simulink model "Half_car_model_susp_bump_tyre"  (R2025b)
settings: Solver=VariableStepAuto  StartTime=0.0  StopTime=10.0  RelTol=1e-3
undefined symbols (not defined in the file or in its folder): bump_t_dist, delta0, Ks, p, r0, u0, x0, x0_lin
libraries: simulink x1

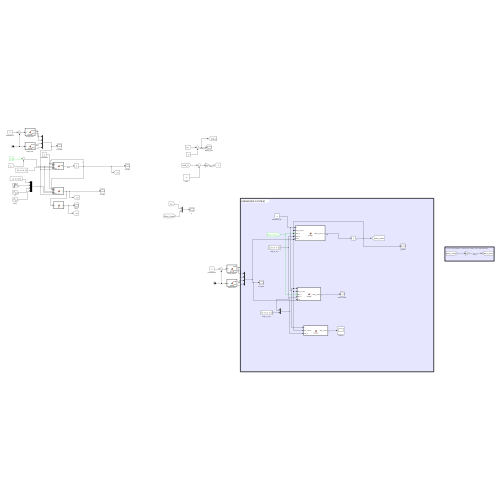
[thumbnail: Simulink's stored preview of the top-level diagram]
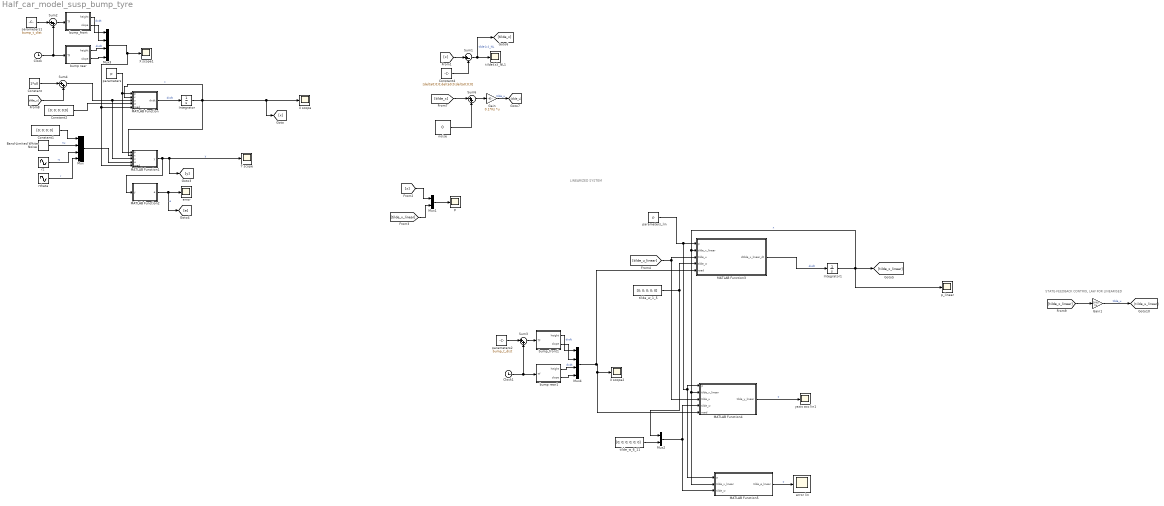
== system Half_car_model_susp_bump_tyre ==
  note: LINEARIZED SYSTEM
  note: STATE-FEEDBACK CONTROL LAW FOR LINEARISED
  " error lin" : Scope
      settings: ActiveDisplayYMinimum=-1  ActiveDisplayYMaximum=1  DataLoggingVariableName=ScopeData5
  Band-Limited White Noise : simulink/Sources/Band-Limited White Noise  Cov="1*[0.00001*1e-2; 0.00001*1e-2;  0.00001*1e-2; 0.00001*1e-2; 0.00001*1e-2]"  Ts=1e-2  seed=[23341; 31826; 11111; 81818; 00001]
  Clock : Clock
  Clock1 : Clock
  Constant : Constant  Value=1*u0
  Constant1 : Constant  Value=[0; 0; 0; 0]
  Constant2 : Constant  Value=[0; 0; 0; 0;0]
  Constant4 : Constant  Value=[delta0;0;0;delta0;0;delta0;0;0]
  Gain : Gain  Gain=0.1*Ks  Multiplication=Matrix(K*u)
  Gain1 : Gain  Gain=1*Ks  Multiplication=Matrix(K*u)
  Integrator : Integrator  InitialCondition=x0
  Integrator1 : Integrator  InitialCondition=x0_lin
  MATLAB Function : MATLAB Function  TreatAsAtomicUnit=on
  MATLAB Function1 : MATLAB Function  TreatAsAtomicUnit=on
  MATLAB Function2 : MATLAB Function  TreatAsAtomicUnit=on
  MATLAB Function3 : MATLAB Function  TreatAsAtomicUnit=on
  MATLAB Function4 : MATLAB Function  TreatAsAtomicUnit=on
  MATLAB Function5 : MATLAB Function  TreatAsAtomicUnit=on
  Mux : Mux
  Mux1 : Mux  Inputs=2
  Mux2 : Mux  Inputs=2
  Mux3 : Mux
  Mux4 : Mux
  Sum1 : Sum  Inputs=|+-
  Sum{2..4,6} (4 alike) : Sum  Inputs=|++
  X scope : Scope
      settings: ActiveDisplayYMinimum=-2.9269551656829207  ActiveDisplayYMaximum=2.5364123096854247  DataLoggingVariableName=ScopeData2
  X scope1 : Scope
      settings: ActiveDisplayYMinimum=-0.062253584416077451  ActiveDisplayYMaximum=0.56028225974469714
  X scope2 : Scope
      settings: ActiveDisplayYMinimum=-2.6804502153599614  ActiveDisplayYMaximum=1.9213273662141332  DataLoggingVariableName=ScopeData9
  Y scope : Scope
      settings: ActiveDisplayYMinimum=-4.5656742824498968  ActiveDisplayYMaximum=4.3230780985024841  DataLoggingVariableName=ScopeData3
  bump rear : MATLAB Function  TreatAsAtomicUnit=on
  bump rear1 : MATLAB Function  TreatAsAtomicUnit=on
  bump_front : MATLAB Function  TreatAsAtomicUnit=on
  bump_front1 : MATLAB Function  TreatAsAtomicUnit=on
  "error " : Scope
      settings: ActiveDisplayYMinimum=-0.92138  ActiveDisplayYMaximum=0.76934  DataLoggingVariableName=ScopeData6
  noise : Constant  Value=0
  p : Scope
      settings: ActiveDisplayYMinimum=-2.11909  ActiveDisplayYMaximum=2.06603
  p_linear : Scope
      settings: ActiveDisplayYMinimum=-1.85296  ActiveDisplayYMaximum=0.95967  DataLoggingVariableName=ScopeData7
  parameters : Constant  Value=p
  parameters1 : Constant  Value=bump_t_dist
  parameters2 : Constant  Value=bump_t_dist
  parameters_lin : Constant  Value=p
  rtheta : Sin  Amplitude=0  Bias=r0  Frequency=0  SampleTime=0
  rz : Sin  Amplitude=0  Bias=r0  Frequency=0  SampleTime=0
  tilde_w_1_5 : Constant  Value=[0; 0; 0; 0; 0]
  tilde_w_6_11 : Constant  Value=[0; 0; 0; 0; 0; 0]
  "tilde{x}_NL1" : Scope
      settings: ActiveDisplayYMinimum=-4.93552  ActiveDisplayYMaximum=2.55492  DataLoggingVariableName=ScopeData4
  yaxis acc lin1 : Scope
      settings: ActiveDisplayYMinimum=-1  ActiveDisplayYMaximum=1  DataLoggingVariableName=ScopeData8
  wires:
  bump rear/1(height) -> Mux3/3  "dxdt"
  Clock/1 -> Sum2/2, bump rear/1(Tf)
  bump_front/2(slope) -> Mux3/2
  bump rear/2(slope) -> Mux3/4
  Sum2/1 -> bump_front/1(Tf)
  parameters1/1 -> Sum2/1
  Mux3/1 -> MATLAB Function1/5(road), MATLAB Function/5(road), X scope1/1
  bump_front/1(height) -> Mux3/1  "dxdt"
  Constant/1 -> Sum4/1
  [tilde_u] -> Sum4/2
  Sum4/1 -> MATLAB Function1/3(u), MATLAB Function/3(u)
  Constant2/1 -> MATLAB Function/4(w)
  MATLAB Function/1(dxdt) -> Integrator/1  "dxdt"
  MATLAB Function1/1(y) -> Y scope/1, [y], MATLAB Function2/1(y)  "y"
  Constant1/1 -> Mux/1
  rtheta/1 -> Mux/4  "r"
  parameters/1 -> MATLAB Function1/1(p), MATLAB Function/1(p)
  Band-Limited White Noise/1 -> Mux/2  "nu"
  rz/1 -> Mux/3  "rz"
  Integrator/1 -> MATLAB Function1/2(x), MATLAB Function/2(x), [x], X scope/1  "x"
  Mux/1 -> MATLAB Function1/4(w)
  MATLAB Function2/1(e) -> [e], "error "/1  "e"
  Sum6/1 -> Gain/1
  [tilde_x] -> Sum6/1
  [x] -> Sum1/1
  [x] -> Mux1/1
  Constant4/1 -> Sum1/2
  Sum1/1 -> [tilde_x], "tilde{x}_NL1"/1  "tilde{x}_NL"
  noise/1 -> Sum6/2
  [tilde_x_linear] -> Mux1/2
  Gain/1 -> [tilde_u]  "tilde_u"
  Mux1/1 -> p/1
  [tilde_x_linear] -> Gain1/1
  Mux2/1 -> MATLAB Function4/4(tilde_w), MATLAB Function5/3(tilde_w)
  tilde_w_1_5/1 -> Mux2/1, MATLAB Function3/4(tilde_w)
  MATLAB Function5/1(tilde_e_linear) -> " error lin"/1  "y"
  [tilde_u_linear] -> MATLAB Function4/3(tilde_u), MATLAB Function3/3(tilde_u)
  parameters_lin/1 -> MATLAB Function5/1(p), MATLAB Function4/1(p), MATLAB Function3/1(p)
  Gain1/1 -> [tilde_u_linear]  "tilde_u"
  MATLAB Function4/1(tilde_y_linear) -> yaxis acc lin1/1  "y"
  Integrator1/1 -> p_linear/1, MATLAB Function5/2(tilde_x_linear), MATLAB Function4/2(tilde_x_linear), MATLAB Function3/2(tilde_x_linear), [tilde_x_linear]  "x"
  tilde_w_6_11/1 -> Mux2/2
  MATLAB Function3/1(dtilde_x_linear_dt) -> Integrator1/1  "dxdt"
  Clock1/1 -> Sum3/2, bump rear1/1(Tf)
  bump_front1/1(height) -> Mux4/1  "dxdt"
  parameters2/1 -> Sum3/1
  bump rear1/1(height) -> Mux4/3  "dxdt"
  Sum3/1 -> bump_front1/1(Tf)
  Mux4/1 -> MATLAB Function3/5(road), MATLAB Function4/5(road), X scope2/1
  bump_front1/2(slope) -> Mux4/2
  bump rear1/2(slope) -> Mux4/4

== matlab function Half_car_model_susp_bump_tyre/MATLAB Function1 ==
  data: p input; x input; u input; y output; w input; road input
function y = h(p,x, u, w, road)

%% parameters
m = p(1);      % [kg] mass
k = p(2);    % [N/m] spring stiffness
beta = p(3);   % [N/(m/s)] damper coeff.
ell0 = p(4);   % [m] 0-load lenght
g = p(5);   % [m/s^2] gravity acceleration
df = p(6);     % [m] distance between center of mass and front
dr = p(7);     % [m] distance between center of mass and rear
J = p(8);      % [kg*m^2] Moment of interti
mwf = p(9);     %[kg] massa ruote AV (asse completo)
mwr = p(10);    %[kg] massa ruote AP (asse completo)
ktf = p(11);   %[N/m] rigidezza pneumatici AV (asse)
ktr = p(12);  %[N/m] rigidezza pneumatici AP (asse)
%% state
pz = x(1);        % [m] heigth of the center of mass of the car 
vz = x(2);        % [m/s] speed of the center of mass of the car 
ptheta = x(3);    % [Rad] pitch angle of the car 
vtheta = x(4);    % [Rad/s] angular speed of the car 
hwheelf = x(5);
dhwheelf = x(6);
hwheelr = x(7);
dhwheelr = x(8);
thetaroad_f = road(4); % [Rad]Road height
zroad_f = road(3);     %[Rad]Road slope
thetaroad_r = road(2); 
zroad_r = -road(1);    

%% disturbance
zgsecond = w(1);
alphag_f = w(2);
alphag_r = w(3);
fwfront = w(4);
fwrear = w(5);

%todo: Vedere se servono due disturbi 

%% state evolution
 
s1 = (pz-hwheelf)+df*(sin(ptheta)-sin(thetaroad_f)); % height of front suspension
s3 = (pz-hwheelr)-dr*(sin(ptheta)-sin(thetaroad_r)); % height of rear suspension

s2 = (vz-dhwheelf)+df*(vtheta*cos(ptheta)-thetaroad_f*cos(thetaroad_f)); % height speed of front suspension
s4 = (vz-dhwheelr)-dr*(vtheta*cos(ptheta)-thetaroad_r*cos(thetaroad_r)); % height speed of rear suspension

lf = s1 + ell0;
lr = s3 + ell0;

%% Forze sospensioni & pneumatici
fsf = -k*s1 - beta*s2;      % sospensione anteriore
fsr = -k*s3 - beta*s4;      % sospensione posteriore

ftf =  ktf*(zroad_f - hwheelf); % pneumatico anteriore (no damping)
ftr =  ktr*(zroad_r - hwheelr); % pneumatico posteriore (no damping)

%% Ripartizione attuatori u1,u2 -> forze su body alle estremità
% [faf + far = u1;   df*faf - dr*far = u2]
faf = (u(2) + dr*u(1))/(df + dr);      % forza attuatore anteriore
far = (df*u(1) - u(2))/(df + dr);      % forza attuatore posteriore

%% Dinamica: corpo
f2 = -g + (fsf + fsr + u(1))/m;                                     % acc. verticale
f4 = (df*fsf - dr*fsr + u(2) + fwfront*lf + fwrear*lr)/J;           % pitch

%% Dinamica: ruote (masse non sospese)
% segno: su ruota, verso +z è (forza pneumatico - forza sospensione - attuatore locale)
f_wf = (ftf - fsf - faf)/mwf;   % acc. ruota ant
f_wr = (ftr - fsr - far)/mwr;   % acc. ruota post


zgsecond = w(1);
alphag = w(2);
fwfront = w(3);
fwrear = w(4);
nuy = w(5);
nuz = w(6);
nug = w(7);
nuf = w(8);
nur = w(9);

%% reference
rz = w(10);
rtheta=w(11);


%% output
y = [sin(x(3))*(f2 + g) + cos(x(3)) * ((fwrear + fwfront) / m)+nuy; 
     cos(x(3))*(f2 + g) - sin(x(3)) * ((fwrear + fwfront) / m)+nuz; %se facciamo cosi ci da in condizioni stazionarie Zaxisacc=9.81, se vogliamo il valore negativo mettere "-" davanti a coseno 
     x(4)+nug;
     s1+nuf;
     s3+nur;
     rz;
     rtheta];
end

== matlab function Half_car_model_susp_bump_tyre/MATLAB Function ==
  data: p input; x input; u input; dxdt output; w input; road input
function dxdt = f(p,x,u,w,road)
%% parameters
%% parameters
m = p(1);      % [kg] mass
k = p(2);    % [N/m] spring stiffness
beta = p(3);   % [N/(m/s)] damper coeff.
ell0 = p(4);   % [m] 0-load lenght
g = p(5);   % [m/s^2] gravity acceleration
df = p(6);     % [m] distance between center of mass and front
dr = p(7);     % [m] distance between center of mass and rear
J = p(8);      % [kg*m^2] Moment of interti
mwf = p(9);     %[kg] massa ruote AV (asse completo)
mwr = p(10);    %[kg] massa ruote AP (asse completo)
ktf = p(11);   %[N/m] rigidezza pneumatici AV (asse)
ktr = p(12);  %[N/m] rigidezza pneumatici AP (asse)
%% state
pz = x(1);        % [m] heigth of the center of mass of the car 
vz = x(2);        % [m/s] speed of the center of mass of the car 
ptheta = x(3);    % [Rad] pitch angle of the car 
vtheta = x(4);    % [Rad/s] angular speed of the car 
hwheelf = x(5);
dhwheelf = x(6);
hwheelr = x(7);
dhwheelr = x(8);
thetaroad_f = road(4); % [Rad]Road height
zroad_f = road(3);     %[Rad]Road slope
thetaroad_r = road(2); 
zroad_r = -road(1);    

%% disturbance
zgsecond = w(1);
alphag_f = w(2);
alphag_r = w(3);
fwfront = w(4);
fwrear = w(5);

%todo: Vedere se servono due disturbi 

%% state evolution
 
s1 = (pz-hwheelf)+df*(sin(ptheta)-sin(thetaroad_f)); % height of front suspension
s3 = (pz-hwheelr)-dr*(sin(ptheta)-sin(thetaroad_r)); % height of rear suspension

s2 = (vz-dhwheelf)+df*(vtheta*cos(ptheta)-thetaroad_f*cos(thetaroad_f)); % height speed of front suspension
s4 = (vz-dhwheelr)-dr*(vtheta*cos(ptheta)-thetaroad_r*cos(thetaroad_r)); % height speed of rear suspension

lf = s1 + ell0;
lr = s3 + ell0;

%% Forze sospensioni & pneumatici
fsf = -k*s1 - beta*s2;      % sospensione anteriore
fsr = -k*s3 - beta*s4;      % sospensione posteriore

ftf =  ktf*(zroad_f - hwheelf); % pneumatico anteriore (no damping)
ftr =  ktr*(zroad_r - hwheelr); % pneumatico posteriore (no damping)

%% Ripartizione attuatori u1,u2 -> forze su body alle estremità
% [faf + far = u1;   df*faf - dr*far = u2]
faf = (u(2) + dr*u(1))/(df + dr);      % forza attuatore anteriore
far = (df*u(1) - u(2))/(df + dr);      % forza attuatore posteriore

%% Dinamica: corpo
f2 = -g + (fsf + fsr + u(1))/m;                                     % acc. verticale
f4 = (df*fsf - dr*fsr + u(2) + fwfront*lf + fwrear*lr)/J;           % pitch

%% Dinamica: ruote (masse non sospese)
% segno: su ruota, verso +z è (forza pneumatico - forza sospensione - attuatore locale)
f_wf = (ftf - fsf - faf)/mwf;   % acc. ruota ant
f_wr = (ftr - fsr - far)/mwr;   % acc. ruota post


%f2 = -g + (((-k*(s1-ell0)-beta*s2)+(-k*(s3-ell0)-beta*s4))+u(1))/m; %  con  ell0
%f4 = (df*(-k*(s1-ell0)-beta*s2)-dr*(-k*(s3-ell0)-beta*s4)+u(2)+fwfront*lf+fwrear*lr)/J; %


%f2 = -g + (((-k*(s1)-beta*s2)+(-k*(s3)-beta*s4))+u(1))/m; %  senza ell0
%f4 = (df*(-k*(s1)-beta*s2)-dr*(-k*(s3)-beta*s4)+u(2)+fwfront*lf+fwrear*lr)/J; %

% dxdt = [vz;
%         f2-zgsecond; 
%         x(4);
%         f4;
%         x(6);
%         alphag];
        
dxdt = [ ...
    vz;                   % pz_dot
    f2 - zgsecond;        % vz_dot
    vtheta;               % ptheta_dot
    f4;                   % vtheta_dot
    dhwheelf;                  % zwf_dot
    f_wf;                 % vwf_dot
    dhwheelr;                  % zwr_dot
    f_wr ]                % vwr_dot




end

== matlab function Half_car_model_susp_bump_tyre/MATLAB Function2 ==
  data: y input; e output
function e = E(y)

df = 1;     % [m] distance between center of mass and front
dr = 1;     % [m] distance between center of mass and rear


yy = y(1); % output of h block yaxisacc 
yz = y(2); % output of h block zaxisacc 
yg = y(3); % output of h block gyro
yf = y(4); % output of h block pot. front
yr = y(5); % output of h block pot. rear
 
%% ref
rz = y(6);
rtheta = y(7);

e = [
    (yf*dr+yr*df)/(dr+df)-rz; 
    asin((yy)/(sqrt(yy^2+yz^2)))-rtheta];
end

== matlab function Half_car_model_susp_bump_tyre/MATLAB Function3 ==
  data: p input; tilde_x_linear input; tilde_u input; dtilde_x_linear_dt output; tilde_w input; road input
function dtilde_x_linear_dt = Linear(p,tilde_x_linear,tilde_u,tilde_w, road)



%% parameters

%% parameters
m = p(1);      % [kg] mass
k = p(2);    % [N/m] spring stiffness
beta = p(3);   % [N/(m/s)] damper coeff.
ell0 = p(4);   % [m] 0-load lenght
g = p(5);   % [m/s^2] gravity acceleration
df = p(6);     % [m] distance between center of mass and front
dr = p(7);     % [m] distance between center of mass and rear
J = p(8);      % [kg*m^2] Moment of interti


delta0 = -m*g/(2*k);




B1 = [0,0;
     1/m, 0;
     0,0;
     0, 1/J;
     0,0;
     0,0];

B2 = [0,0,0,0,0;
      -1,0,0,0,0;
      0,0,0,0,0;
      0,0,(delta0+ell0)/J,(delta0+ell0)/J, 0;
      0,0,0,0,0;
      0,1,0,0,0];




%% state evolution
dtilde_x_linear_dt = A*tilde_x_linear+B1*tilde_u+B2*tilde_w;
end

== matlab function Half_car_model_susp_bump_tyre/MATLAB Function4 ==
  data: p input; tilde_x_linear input; tilde_u input; tilde_y_linear output; tilde_w input; road input
function tilde_y_linear = Linear(p,tilde_x_linear,tilde_u,tilde_w, road)


%% parameters
m = p(1);      % [kg] mass
k = p(2);    % [N/m] spring stiffness
beta = p(3);   % [N/(m/s)] damper coeff.
ell0 = p(4);   % [m] 0-load lenght
g = p(5);   % [m/s^2] gravity acceleration
df = p(6);     % [m] distance between center of mass and front
dr = p(7);     % [m] distance between center of mass and rear
J = p(8);      % [kg*m^2] Moment of interti



C = [0, 0, g, 0, 0, 0;
    -2*k/m, -2*beta/m, -k*(df-dr)/m, -beta*(df-dr)/m, k*(df-dr)/m, beta*(df-dr)/m;
    0, 0, 0, 1, 0, 0;
    1, 0, df, 0, -df, 0;
    1, 0, -dr, 0, dr, 0];


D1 = [0,0;
     1/m, 0;
     0,0;
     0,0;
     0,0];

D2 = [0,0,1/m,1/m,1,0,0,0,0,0,0;
      0,0,0,0,0,1,0,0,0,0,0;
      0,0,0,0,0,0,1,0,0,0,0;
      0,0,0,0,0,0,0,1,0,0,0;
      0,0,0,0,0,0,0,0,1,0,0];




%% state evolution
tilde_y_linear = C*tilde_x_linear+D1*tilde_u+D2*tilde_w;
end

== matlab function Half_car_model_susp_bump_tyre/MATLAB Function5 ==
  data: p input; tilde_x_linear input; tilde_e_linear output; tilde_w input
function tilde_e_linear = Linear(p,tilde_x_linear,tilde_w)


%% parameters
m = p(1);      % [kg] mass
k = p(2);    % [N/m] spring stiffness
beta = p(3);   % [N/(m/s)] damper coeff.
ell0 = p(4);   % [m] 0-load lenght
g = p(5);   % [m/s^2] gravity acceleration
df = p(6);     % [m] distance between center of mass and front
dr = p(7);     % [m] distance between center of mass and rear
J = p(8);      % [kg*m^2] Moment of interti



Ce = [1,0,0,0,0,0;
      0,0,1,0,0,0];



De2 = [0,0,0,0,0,0,0,dr/(dr+df),df/(dr+df),-1,0;
       0,0, 1/(m*g),1/(m*g),1/g,0,0,0,0,0,-1];




%% state evolution
tilde_e_linear = Ce*tilde_x_linear+De2*tilde_w;
end

== matlab function Half_car_model_susp_bump_tyre/bump rear ==
  data: height output; slope output; Tf input
function [height, slope] = bump(Tf)
    % Parametri
    a = 0.1;       % Ampiezza del bump (m)
    V = 20;         % Velocità del veicolo (m/s)
    lambda = 5;     % Lunghezza dell'onda del bump (m)
    Tspan = 5;      % Durata della simulazione (s)
    T1 = 5;         % Tempo di inizio del bump
    T2 = T1 + lambda/V; % Tempo di fine del bump

    % Calcola l'altezza della strada in base alla funzione del bump
    % Sostituzione di heaviside con un controllo manuale
    height = (a/2) * (1 - cos((2*pi*V*Tf)/lambda)) .* (Tf >= T1 & Tf <= T2); 
    
    % Calcola la pendenza della strada (derivata prima dell'altezza rispetto al tempo)
    slope = (a/2) * (2*pi*V/lambda) .* sin((2*pi*V*Tf)/lambda) .* (Tf >= T1 & Tf <= T2); 
end

== matlab function Half_car_model_susp_bump_tyre/bump_front ==
  data: height output; slope output; Tf input
function [height, slope] = bump(Tf)
    % Parametri
    a = 0.1;       % Ampiezza del bump (m)
    V = 20;         % Velocità del veicolo (m/s)
    lambda = 5;     % Lunghezza dell'onda del bump (m)
    Tspan = 5;      % Durata della simulazione (s)
    T1 = 5;         % Tempo di inizio del bump
    T2 = T1 + lambda/V; % Tempo di fine del bump

    % Calcola l'altezza della strada in base alla funzione del bump
    % Sostituzione di heaviside con un controllo manuale
    height = (a/2) * (1 - cos((2*pi*V*Tf)/lambda)) .* (Tf >= T1 & Tf <= T2); 
    
    % Calcola la pendenza della strada (derivata prima dell'altezza rispetto al tempo)
    slope = (a/2) * (2*pi*V/lambda) .* sin((2*pi*V*Tf)/lambda) .* (Tf >= T1 & Tf <= T2); 
end

== matlab function Half_car_model_susp_bump_tyre/bump rear1 ==
  data: height output; slope output; Tf input
function [height, slope] = bump(Tf)
    % Parametri
    a = 0.1;       % Ampiezza del bump (m)
    V = 20;         % Velocità del veicolo (m/s)
    lambda = 5;     % Lunghezza dell'onda del bump (m)
    Tspan = 5;      % Durata della simulazione (s)
    T1 = 5;         % Tempo di inizio del bump
    T2 = T1 + lambda/V; % Tempo di fine del bump

    % Calcola l'altezza della strada in base alla funzione del bump
    % Sostituzione di heaviside con un controllo manuale
    height = (a/2) * (1 - cos((2*pi*V*Tf)/lambda)) .* (Tf >= T1 & Tf <= T2); 
    
    % Calcola la pendenza della strada (derivata prima dell'altezza rispetto al tempo)
    slope = (a/2) * (2*pi*V/lambda) .* sin((2*pi*V*Tf)/lambda) .* (Tf >= T1 & Tf <= T2); 
end

== matlab function Half_car_model_susp_bump_tyre/bump_front1 ==
  data: height output; slope output; Tf input
function [height, slope] = bump(Tf)
    % Parametri
    a = 0.1;       % Ampiezza del bump (m)
    V = 20;         % Velocità del veicolo (m/s)
    lambda = 5;     % Lunghezza dell'onda del bump (m)
    Tspan = 5;      % Durata della simulazione (s)
    T1 = 5;         % Tempo di inizio del bump
    T2 = T1 + lambda/V; % Tempo di fine del bump

    % Calcola l'altezza della strada in base alla funzione del bump
    % Sostituzione di heaviside con un controllo manuale
    height = (a/2) * (1 - cos((2*pi*V*Tf)/lambda)) .* (Tf >= T1 & Tf <= T2); 
    
    % Calcola la pendenza della strada (derivata prima dell'altezza rispetto al tempo)
    slope = (a/2) * (2*pi*V/lambda) .* sin((2*pi*V*Tf)/lambda) .* (Tf >= T1 & Tf <= T2); 
end
